simulink model "MODEL"  (R2024b)
settings: Solver=FixedStepAuto  StartTime=0.0  StopTime=10  FixedStep=0.0001  RelTol=1e-3
libraries: commseqgen3 x4, dspfdesign x2
settings Model: Creator=ET  LastModifiedBy=anwithavishwanath
settings DebuggingCC: ParameterPrecisionLossMsg=none  UnconnectedInputMsg=warning  UnconnectedOutputMsg=warning  UnconnectedLineMsg=warning
settings ModelReferenceCC: EnableRefExpFcnMdlSchedulingChecks=on
settings RTWCC: RTWVerbose=off  GPUComputeCapability=3.5  DLArmComputeVersion=19.05

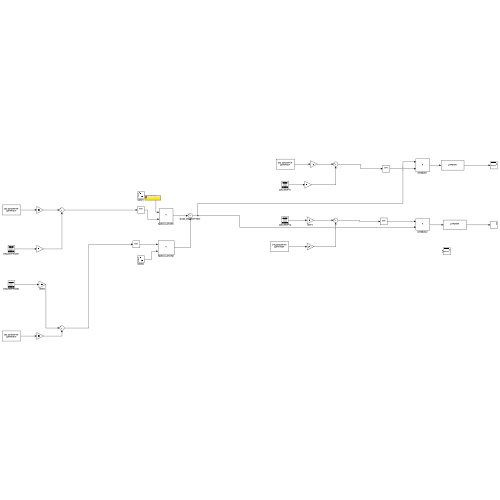
[thumbnail: Simulink's stored preview of the top-level diagram]
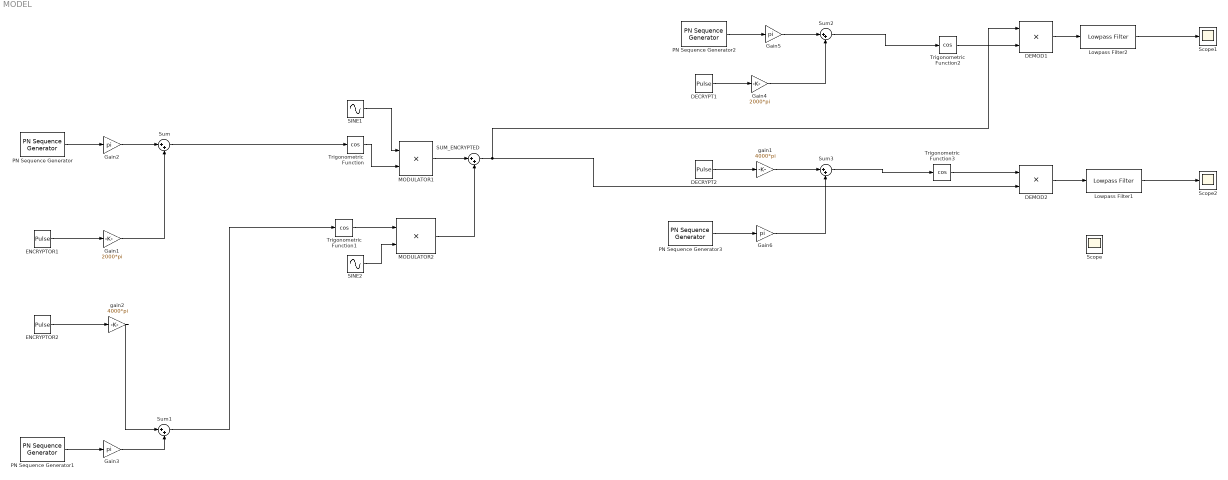
== system MODEL ==
  DECRYPT1 : DiscretePulseGenerator  Period=10  PulseWidth=5  SampleTime=0.0001
  DECRYPT2 : DiscretePulseGenerator  Period=10  PulseWidth=5  SampleTime=0.0001
  DEMOD1 : Product
  DEMOD2 : Product
  ENCRYPTOR1 : DiscretePulseGenerator  Period=10  PulseWidth=5  SampleTime=0.0001
  ENCRYPTOR2 : DiscretePulseGenerator  Period=5  PulseWidth=3  SampleTime=0.0001
  Gain1 : Gain  Gain=2000*pi
  Gain{2..3,5..6} (4 alike) : Gain  Gain=pi
  Gain4 : Gain  Gain=2000*pi
  Lowpass Filter1 : dspfdesign/Lowpass Filter  FilterType=FIR  DesignForMinimumOrder=off  FilterOrder=50  PassbandFrequency=0.003  StopbandFrequency=0.5442  PassbandRipple=1  StopbandAttenuation=60  SampleRateMode=Specify on dialog  SampleRate=10000  SimulateUsing=Interpreted execution  roundingMode=Floor  coeffsDataTypeStr=fixdt(1,16)
  Lowpass Filter2 : dspfdesign/Lowpass Filter  FilterType=FIR  DesignForMinimumOrder=off  FilterOrder=50  PassbandFrequency=0.0015  StopbandFrequency=0.5442  PassbandRipple=1  StopbandAttenuation=60  SampleRateMode=Specify on dialog  SampleRate=10000  SimulateUsing=Interpreted execution  roundingMode=Floor  coeffsDataTypeStr=fixdt(1,16)
  MODULATOR1 : Product
  MODULATOR2 : Product
  PN Sequence Generator{,1..3} (4 alike) : commseqgen3/PN Sequence Generator  poly='z^6 + z + 1'  ini_sta=[0 0 0 0 0 1]  outBitMaskSource=Dialog parameter  shift=0  outVarSiz=off  maxOutSizeMode=Dialog parameter  maxOutSize=[10 1]  Ts=0.0001  sampPerFrame=1  reset=off  bitPackedOutputs=off  outDataType=boolean  numPackedBits=8  bitPackDataSigned=off  bitPackedOutDType=double
  SINE1 : Sin  SineType=Sample based  Frequency=10  Samples=1000  SampleTime=0.0001
  SINE2 : Sin  SineType=Sample based  Frequency=20  Samples=500  SampleTime=0.0001
  SUM_ENCRYPTED : Sum  Inputs=|++
  Scope : Scope
  Scope1 : Scope
  Scope2 : Scope
  Sum{,1..3} (4 alike) : Sum  Inputs=|++
  Trigonometric Function{,1..3} (4 alike) : Trigonometry  Operator=cos
  gain1 : Gain  Gain=4000*pi
  gain2 : Gain  Gain=4000*pi
  wires:
  PN Sequence Generator/1 -> Gain2/1
  PN Sequence Generator1/1 -> Gain3/1
  Gain2/1 -> Sum/1
  Gain1/1 -> Sum/2
  gain2/1 -> Sum1/1
  Gain3/1 -> Sum1/2
  Sum/1 -> Trigonometric Function/1
  Sum1/1 -> Trigonometric Function1/1
  SINE1/1 -> MODULATOR1/1
  Trigonometric Function/1 -> MODULATOR1/2
  Trigonometric Function1/1 -> MODULATOR2/1
  SINE2/1 -> MODULATOR2/2
  MODULATOR1/1 -> SUM_ENCRYPTED/1
  MODULATOR2/1 -> SUM_ENCRYPTED/2
  SUM_ENCRYPTED/1 -> DEMOD1/1, DEMOD2/2
  Gain5/1 -> Sum2/1
  PN Sequence Generator3/1 -> Gain6/1
  gain1/1 -> Sum3/1
  Gain4/1 -> Sum2/2
  Gain6/1 -> Sum3/2
  PN Sequence Generator2/1 -> Gain5/1
  Sum2/1 -> Trigonometric Function2/1
  Sum3/1 -> Trigonometric Function3/1
  Trigonometric Function2/1 -> DEMOD1/2
  Trigonometric Function3/1 -> DEMOD2/1
  DEMOD1/1 -> Lowpass Filter2/1
  DEMOD2/1 -> Lowpass Filter1/1
  Lowpass Filter2/1 -> Scope1/1
  ENCRYPTOR2/1 -> gain2/1
  ENCRYPTOR1/1 -> Gain1/1
  DECRYPT1/1 -> Gain4/1
  DECRYPT2/1 -> gain1/1
  Lowpass Filter1/1 -> Scope2/1
